simulink model "ThreeMotorModelSimulationX_PIDTESTNG"  (R2020b)
settings: Solver=ode14x  StartTime=0.0  StopTime=SimTime  FixedStep=SimStepTime  RelTol=1e-3
InitFcn:
  | StartupScript
StartFcn:
  | StartupScript
values from neighbouring files (symbols this model uses):
  CF = 372.0    (= 372)    [StartupScript.m]
  d2r = pi/180    (= 0.0174532925199)    [StartupScript.m]
  Isat = 10.0    (= 10)    [StartupScript.m]
  Ka = 1    [StartupScript.m]
  Kb = 1    [StartupScript.m]
  Kda = 50    [StartupScript.m]
  Kdb = 280    [StartupScript.m]
  Kdr = 3.4    [StartupScript.m]
  Kia = 150    [StartupScript.m]
  Kib = 200    [StartupScript.m]
  Kir = 6.1    [StartupScript.m]
  Kma = 19.5*1e-3    (= 0.0195)    [StartupScript.m]
  Kmb = 23.4*1e-3    (= 0.0234)    [StartupScript.m]
  Kmr = 29.9*1e-3    (= 0.0299)    [StartupScript.m]
  Kpa = 1250    [StartupScript.m]
  Kpb = 1500    [StartupScript.m]
  Kpr = 40    [StartupScript.m]
  Kr = 1    [StartupScript.m]
  PidLim = 1024    [StartupScript.m]
  PidUCGain = 5/1024    (= 0.0048828125)    [StartupScript.m]
  r2d = 180/pi    (= 57.2957795131)    [StartupScript.m]
  sensorGain = 1/1024.0    (= 0.0009765625)    [StartupScript.m]
  SimStepTime = 1e-3    (= 0.001)    [StartupScript.m]
  Vsat = 24.0    (= 24)    [StartupScript.m]
libraries: cstblocks x9, simulink x1
settings Model: Creator=nisch  LastModifiedBy=nisch

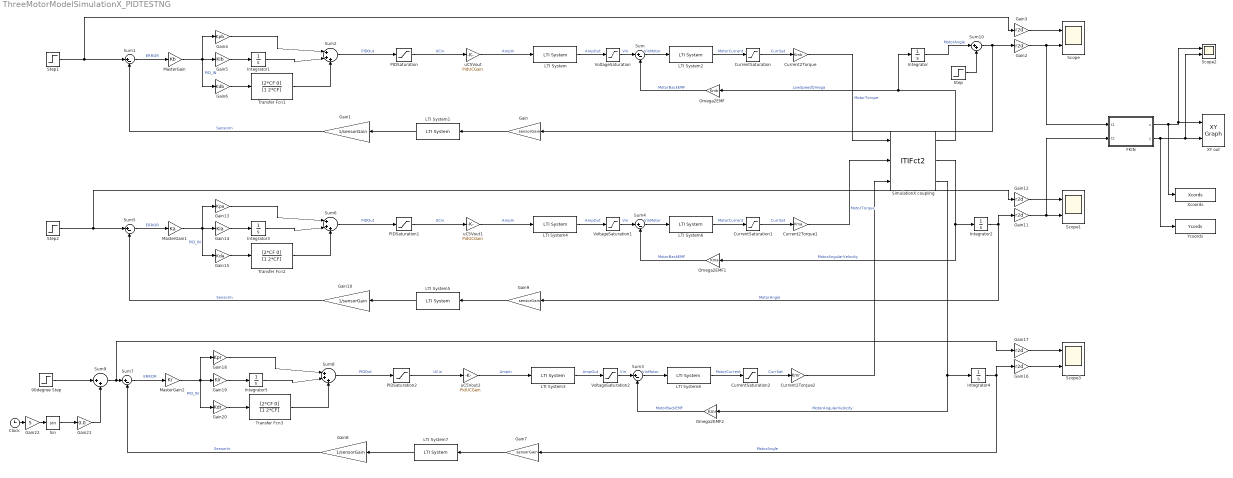
== system ThreeMotorModelSimulationX_PIDTESTNG ==
  90degree Step : Step  Time=0  After=180*d2r  SampleTime=0
  Clock : Clock
  Current2Torque : Gain  Gain=Kmb
  Current2Torque1 : Gain  Gain=Kma
  Current2Torque2 : Gain  Gain=Kmr
  CurrentSaturation : Saturate  UpperLimit=Isat  LowerLimit=-Isat
  CurrentSaturation1 : Saturate  UpperLimit=Isat  LowerLimit=-Isat
  CurrentSaturation2 : Saturate  UpperLimit=Isat  LowerLimit=-Isat
  FKIN : MATLAB Function  TreatAsAtomicUnit=on
  Gain : Gain  Gain=sensorGain
  Gain1 : Gain  Gain=1/sensorGain
  Gain10 : Gain  Gain=1/sensorGain
  Gain{2..3,11..12,16..17} (6 alike) : Gain  Gain=r2d
  Gain13 : Gain  Gain=Kpa
  Gain14 : Gain  Gain=Kia
  Gain15 : Gain  Gain=Kda
  Gain18 : Gain  Gain=Kpr
  Gain19 : Gain  Gain=Kir
  Gain20 : Gain  Gain=Kdr
  Gain21 : Gain  Gain=0.0
  Gain22 : Gain  Gain=5
  Gain4 : Gain  Gain=Kpb
  Gain5 : Gain  Gain=Kib
  Gain6 : Gain  Gain=Kdb
  Gain7 : Gain  Gain=sensorGain
  Gain8 : Gain  Gain=1/sensorGain
  Gain9 : Gain  Gain=sensorGain
  Integrator{,1..5} (6 alike) : Integrator
  LTI System : cstblocks/LTI System  sys=VoltageAmplifier  IC=[]
  LTI System1 : cstblocks/LTI System  sys=Hs  IC=[]
  LTI System2 : cstblocks/LTI System  sys=Electricalb  IC=[]
  LTI System3 : cstblocks/LTI System  sys=VoltageAmplifier  IC=[]
  LTI System4 : cstblocks/LTI System  sys=VoltageAmplifier  IC=[]
  LTI System5 : cstblocks/LTI System  sys=Hs  IC=[]
  LTI System6 : cstblocks/LTI System  sys=Electricala  IC=[]
  LTI System7 : cstblocks/LTI System  sys=Hs  IC=[]
  LTI System8 : cstblocks/LTI System  sys=Electricalr  IC=[]
  MasterGain : Gain  Gain=Kb
  MasterGain1 : Gain  Gain=Ka
  MasterGain2 : Gain  Gain=Kr
  Omega2EMF : Gain  Gain=Kmb
  Omega2EMF1 : Gain  Gain=Kma
  Omega2EMF2 : Gain  Gain=Kmr
  PIDSaturation : Saturate  UpperLimit=PidLim  LowerLimit=-PidLim
  PIDSaturation1 : Saturate  UpperLimit=PidLim  LowerLimit=-PidLim
  PIDSaturation2 : Saturate  UpperLimit=PidLim  LowerLimit=-PidLim
  Scope{,1..3} (4 alike) : Scope  NumInputPorts=2
  SimulationX coupling : S-Function  FunctionName=ITIFct2  Parameters=ip, port, ts, nIn, nOut  SFunctionDeploymentMode=off  EnableBusSupport=off  mask{ip='localhost', port=4097, ts=SimStepTime, nIn=3, nOut=3}
      mask prompts: ip "Address: ip"; port "Port Number: port [-]"; ts "Communication Step Size: ts [s]"; nIn "Input Vector Dimension (to SimulationX): nIn [-]"; nOut "Output Vector Dimension (from SimulationX): nOut [-]"
      mask help: Coupling Element
  Sin : Trigonometry
  Step : Step  Time=0  After=30*d2r  SampleTime=0
  Step1 : Step  Time=0  After=120*d2r  SampleTime=0
  Step2 : Step  Time=0  After=0*d2r  SampleTime=0
  Sum{,1,3..5,7} (6 alike) : Sum  Inputs=|+-
  Sum10 : Sum  Inputs=|++
  Sum2 : Sum  Inputs=|+++
  Sum6 : Sum  Inputs=|+++
  Sum8 : Sum  Inputs=|+++
  Sum9 : Sum  Inputs=|++
  Transfer Fcn1 : TransferFcn  Numerator=[2*CF 0]  Denominator=[1 2*CF]
  Transfer Fcn2 : TransferFcn  Numerator=[2*CF 0]  Denominator=[1 2*CF]
  Transfer Fcn3 : TransferFcn  Numerator=[2*CF 0]  Denominator=[1 2*CF]
  VoltageSaturation : Saturate  UpperLimit=Vsat  LowerLimit=-Vsat
  VoltageSaturation1 : Saturate  UpperLimit=Vsat  LowerLimit=-Vsat
  VoltageSaturation2 : Saturate  UpperLimit=Vsat  LowerLimit=-Vsat
  XY out : simulink/Sinks/XY Graph  xmin=-50  xmax=50  ymin=-50  ymax=50  st=-1
  Xcoords : ToWorkspace  VariableName=Xcords  SaveFormat=Timeseries  SampleTime=-1
  Ycoords : ToWorkspace  VariableName=Ycords  SaveFormat=Timeseries  SampleTime=-1
  uC5Vout : Gain  Gain=PidUCGain
  uC5Vout1 : Gain  Gain=PidUCGain
  uC5Vout2 : Gain  Gain=PidUCGain
  wires:
  LTI System/1 -> VoltageSaturation/1  "AmpOut"
  PIDSaturation/1 -> uC5Vout/1  "UCin"
  VoltageSaturation/1 -> Sum/1  "Vin"
  uC5Vout/1 -> LTI System/1  "AmpIn"
  Gain/1 -> LTI System1/1
  Gain6/1 -> Transfer Fcn1/1
  Gain5/1 -> Integrator1/1
  Sum1/1 -> MasterGain/1  "ERROR"
  LTI System2/1 -> CurrentSaturation/1  "MotorCurrent"
  CurrentSaturation/1 -> Current2Torque/1  "CurrSat"
  Gain2/1 -> FKIN/1(t1), Scope/2
  Transfer Fcn1/1 -> Sum2/3
  Sum/1 -> LTI System2/1  "VinMotor"
  Gain4/1 -> Sum2/1
  Integrator1/1 -> Sum2/2
  MasterGain/1 -> Gain6/1, Gain5/1, Gain4/1  "PID_IN"
  Sum2/1 -> PIDSaturation/1  "PIDOut"
  Omega2EMF/1 -> Sum/2  "MotorBackEMF"
  LTI System1/1 -> Gain1/1
  Gain1/1 -> Sum1/2  "SensorIn"
  Gain3/1 -> Scope/1
  Gain9/1 -> LTI System5/1
  Gain11/1 -> Scope1/2, FKIN/2(t2)
  VoltageSaturation1/1 -> Sum4/1  "Vin"
  PIDSaturation1/1 -> uC5Vout1/1  "UCin"
  LTI System5/1 -> Gain10/1
  LTI System4/1 -> VoltageSaturation1/1  "AmpOut"
  SimulationX coupling/2 -> Omega2EMF1/1, Integrator2/1  "MotorAngularVelocity"
  LTI System6/1 -> CurrentSaturation1/1  "MotorCurrent"
  Gain15/1 -> Transfer Fcn2/1
  CurrentSaturation1/1 -> Current2Torque1/1  "CurrSat"
  Gain14/1 -> Integrator3/1
  Omega2EMF1/1 -> Sum4/2  "MotorBackEMF"
  Sum6/1 -> PIDSaturation1/1  "PIDOut"
  MasterGain1/1 -> Gain15/1, Gain14/1, Gain13/1  "PID_IN"
  uC5Vout1/1 -> LTI System4/1  "AmpIn"
  Integrator3/1 -> Sum6/2
  Sum4/1 -> LTI System6/1  "VinMotor"
  Transfer Fcn2/1 -> Sum6/3
  Integrator2/1 -> Gain11/1, Gain9/1  "MotorAngle"
  Gain13/1 -> Sum6/1
  Gain12/1 -> Scope1/1
  Sum5/1 -> MasterGain1/1  "ERROR"
  Gain10/1 -> Sum5/2  "SensorIn"
  FKIN/1(x) -> Xcoords/1, XY out/1, Scope2/1
  FKIN/2(y) -> XY out/2, Scope2/2, Ycoords/1
  SimulationX coupling/1 -> Omega2EMF/1, Integrator/1  "LowSpeedOmega"
  Current2Torque/1 -> SimulationX coupling/1  "MotorTorque"
  Current2Torque1/1 -> SimulationX coupling/2  "MotorTorque"
  Sum8/1 -> PIDSaturation2/1  "PIDOut"
  Gain7/1 -> LTI System7/1
  Gain20/1 -> Transfer Fcn3/1
  Gain17/1 -> Scope3/1
  uC5Vout2/1 -> LTI System3/1  "AmpIn"
  Omega2EMF2/1 -> Sum3/2  "MotorBackEMF"
  Sum3/1 -> LTI System8/1  "VinMotor"
  MasterGain2/1 -> Gain20/1, Gain19/1, Gain18/1  "PID_IN"
  CurrentSaturation2/1 -> Current2Torque2/1  "CurrSat"
  90degree Step/1 -> Sum9/1
  Gain18/1 -> Sum8/1
  Clock/1 -> Gain22/1
  Sum9/1 -> Gain17/1, Sum7/1
  Gain22/1 -> Sin/1
  LTI System8/1 -> CurrentSaturation2/1  "MotorCurrent"
  Gain19/1 -> Integrator5/1
  Integrator5/1 -> Sum8/2
  VoltageSaturation2/1 -> Sum3/1  "Vin"
  Transfer Fcn3/1 -> Sum8/3
  Sin/1 -> Gain21/1
  Gain8/1 -> Sum7/2  "SensorIn"
  PIDSaturation2/1 -> uC5Vout2/1  "UCin"
  LTI System7/1 -> Gain8/1
  LTI System3/1 -> VoltageSaturation2/1  "AmpOut"
  SimulationX coupling/3 -> Omega2EMF2/1, Integrator4/1  "MotorAngularVelocity"
  Gain21/1 -> Sum9/2
  Sum7/1 -> MasterGain2/1  "ERROR"
  Gain16/1 -> Scope3/2
  Integrator4/1 -> Gain16/1, Gain7/1  "MotorAngle"
  Current2Torque2/1 -> SimulationX coupling/3
  Integrator/1 -> Sum10/1  "MotorAngle"
  Sum10/1 -> Gain/1, Gain2/1
  Step/1 -> Sum10/2
  Step1/1 -> Sum1/1, Gain3/1
  Step2/1 -> Sum5/1, Gain12/1

== matlab function ThreeMotorModelSimulationX_PIDTESTNG/FKIN ==
  data: t1 input; x output; t2 input; y output
function [x, y] = ForwardKin(t1, t2)
    
    Larm1 = 30;
    Larm2 = 15;
    
    arm1X = Larm1 * cos(t1*pi/180);
    arm1Y = Larm1 * sin(t1*pi/180);

    arm2X = Larm2 * cos((t2+t1)*pi/180) + arm1X;
    arm2Y = Larm2 * sin((t2+t1)*pi/180) + arm1Y;
    
    y = arm2Y;
    x = arm2X;
end
